simulink model "sgp4_test"  (R2018b)
settings: Solver=VariableStepAuto  StartTime=0.0  StopTime=7304  RelTol=1e-3
undefined symbols (not defined in the file or in its folder): simParams
libraries: sgp4_lib_fsw x1
settings Model: Creator=colem  LastModifiedBy=taylorreynolds

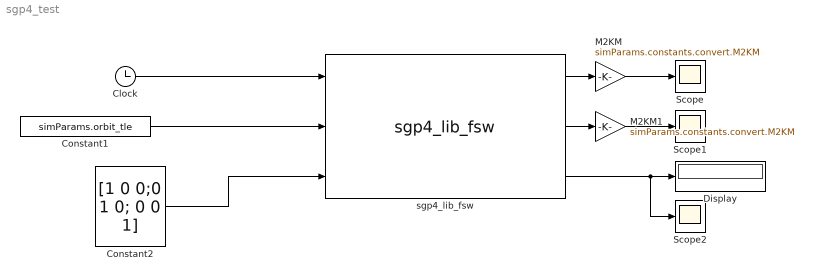
== system sgp4_test ==
  Clock : Clock
  Constant1 : Constant  Value=simParams.orbit_tle
  Constant2 : Constant  Value=[1 0 0;0 1 0; 0 0 1]
  Display : Display
  M2KM : Gain  Gain=simParams.constants.convert.M2KM
  M2KM1 : Gain  Gain=simParams.constants.convert.M2KM
  Scope : Scope
  Scope1 : Scope
  Scope2 : Scope
  sgp4_lib_fsw : sgp4_lib_fsw/sgp4_lib_fsw  SystemSampleTime=-1
  wires:
  Constant1/1 -> sgp4_lib_fsw/2
  Constant2/1 -> sgp4_lib_fsw/3
  sgp4_lib_fsw/1 -> M2KM/1
  sgp4_lib_fsw/2 -> M2KM1/1
  sgp4_lib_fsw/3 -> Scope2/1, Display/1
  Clock/1 -> sgp4_lib_fsw/1
  M2KM/1 -> Scope/1
  M2KM1/1 -> Scope1/1
